simulink model "PIPID_Control"  (R2018a)
settings: Solver=ode5  StartTime=0.0  StopTime=70  FixedStep=0.001  RelTol=1e-3
settings Model: Creator=Yinan  LastModifiedBy=Yinan

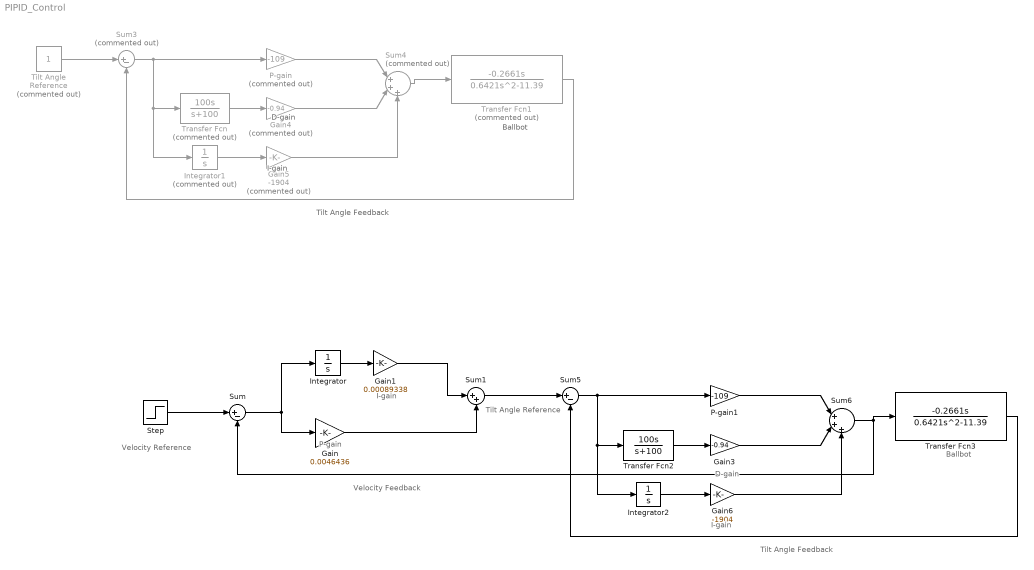
== system PIPID_Control ==
  note: Tilt Angle Reference
  note: Velocity Feedback
  note: Velocity Reference
  note: P-gain
  note: I-gain
  note: I-gain
  note: D-gain
  note: Ballbot
  note: Tilt Angle Feedback
  note: D-gain
  note: I-gain
  note: Ballbot
  note: Tilt Angle Feedback
  Gain : Gain  Gain=0.0046436
  Gain1 : Gain  Gain=0.00089338
  Gain3 : Gain  Gain=-0.94
  Gain4 : Gain  Commented=on  Gain=-0.94
  Gain5 : Gain  Commented=on  Gain=-1904
  Gain6 : Gain  Gain=-1904
  Integrator : Integrator
  Integrator1 : Integrator  Commented=on
  Integrator2 : Integrator
  P-gain : Gain  Commented=on  Gain=-109
  P-gain1 : Gain  Gain=-109
  Step : Step  After=20  SampleTime=0
  Sum : Sum  Inputs=|+-
  Sum1 : Sum  Inputs=|++
  Sum3 : Sum  Commented=on  Inputs=|+-
  Sum4 : Sum  Commented=on  Inputs=|+++
  Sum5 : Sum  Inputs=|+-
  Sum6 : Sum  Inputs=|+++
  Tilt Angle Reference : Constant  Commented=on
  Transfer Fcn : TransferFcn  Commented=on  Numerator=[100 0]  Denominator=[1 100]
  Transfer Fcn1 : TransferFcn  Commented=on  Numerator=[-0.2661 0]  Denominator=[0.6421 0 -11.39]
  Transfer Fcn2 : TransferFcn  Numerator=[100 0]  Denominator=[1 100]
  Transfer Fcn3 : TransferFcn  Numerator=[-0.2661 0]  Denominator=[0.6421 0 -11.39]
  wires:
  Sum3/1 -> Transfer Fcn/1, Integrator1/1, P-gain/1
  Transfer Fcn/1 -> Gain4/1
  P-gain/1 -> Sum4/1
  Gain4/1 -> Sum4/2
  Tilt Angle Reference/1 -> Sum3/1
  Sum4/1 -> Transfer Fcn1/1
  Transfer Fcn1/1 -> Sum3/2
  Integrator1/1 -> Gain5/1
  Gain5/1 -> Sum4/3
  Sum6/1 -> Transfer Fcn3/1, Sum/2
  Gain6/1 -> Sum6/3
  Transfer Fcn3/1 -> Sum5/2
  Integrator2/1 -> Gain6/1
  Transfer Fcn2/1 -> Gain3/1
  P-gain1/1 -> Sum6/1
  Gain3/1 -> Sum6/2
  Sum5/1 -> Transfer Fcn2/1, Integrator2/1, P-gain1/1
  Sum1/1 -> Sum5/1
  Sum/1 -> Integrator/1, Gain/1
  Integrator/1 -> Gain1/1
  Gain/1 -> Sum1/2
  Step/1 -> Sum/1
  Gain1/1 -> Sum1/1
